simulink model "lab07"  (Simulink 10.3)
settings: Solver=FixedStepAuto  StartTime=0.0  StopTime=2.5  FixedStep=0.001768  RelTol=1e-3
values from neighbouring files (symbols this model uses):
  D = 0    [lab03.mat]    (also in lab04.mat; lab05.mat; lab07.mat; matlab.mat)
  k_d = 0.00416035381008    [lab03.mat]    (also in lab04.mat = 0.00114359359927; lab05.mat = 0.00883154670201; lab06.mat = 0.05; lab07.mat = 0.00883154670201)
  k_p = 2    [lab02.mat]    (also in lab03.mat = 0.256097247605; lab04.mat = 0.137612608424; lab05.mat = 0.280842058008; lab06.mat = 0.012)
undefined symbols (not defined in the file or in its folder): D_n, N_1, N_2, N_n
settings Model: Creator=kisdev  LastModifiedBy=kisdev
settings SolverCC: AlgebraicLoopSolver=Auto
settings DataIOCC: SaveFormat=Dataset  SignalLoggingSaveFormat=Dataset  ReturnWorkspaceOutputs=on
settings OptimizationCC: ExpressionDepthLimit=128  LifeSpan=auto
settings DebuggingCC: UnderspecifiedInitializationDetection=Simplified  MergeDetectMultiDrivingBlocksExec=error  FcnCallInpInsideContextMsg=error  StateNameClashWarn=none  SFUnexpectedBacktrackingDiag=error  SFNoUnconditionalDefaultTransitionDiag=error  SFExecutionAtInitializationDiag=warning  SFMachineParentedDataDiag=error  ArithmeticOperatorsInVariantConditions=error
settings HardwareCC: ProdBitPerPointer=64  ProdBitPerSizeT=64  ProdBitPerPtrDiffT=64  ProdLargestAtomicFloat=Float  ProdIntDivRoundTo=Zero  ProdEndianess=LittleEndian  ProdWordSize=64  ProdHWDeviceType=Intel->x86-64 (Windows64)
settings ModelReferenceCC: PropagateSignalLabelsOutOfModel=on
settings SFSimCC: SimUseLocalCustomCode=on  CustomCodeUndefinedFunction=FilterOut
settings RTWCC: RTWUseLocalCustomCode=on
settings CodeAppCC: StateflowObjectComments=off
settings GRTTargetCC: TargetLangStandard=C99 (ISO)  CombineOutputUpdateFcns=on  GRTInterface=off
settings ConfigComp: CovMetricSettings=dwe  CovSaveCumulativeToWorkspaceVar=off  CovSaveSingleToWorkspaceVar=off  CovExternalEMLEnable=on

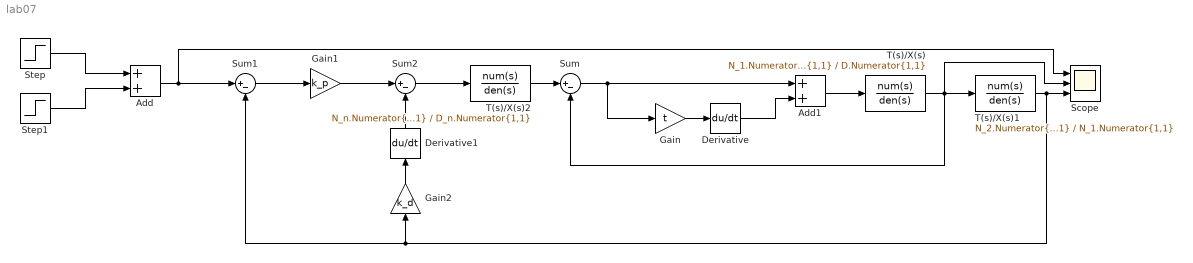
== system lab07 ==
  Add : Sum
  Add1 : Sum
  Derivative : Derivative
  Derivative1 : Derivative
  Gain : Gain  Gain=t
  Gain1 : Gain  Gain=k_p
  Gain2 : Gain  Gain=k_d
  Scope : Scope  NumInputPorts=3
  Step : Step  Time=0  After=500  SampleTime=0
  Step1 : Step  Time=10  After=-500  SampleTime=0
  Sum : Sum  Inputs=|+-
  Sum1 : Sum  Inputs=|+-
  Sum2 : Sum  Inputs=|+-
  T(s)/X(s) : TransferFcn  Numerator=N_1.Numerator{1,1}  Denominator=D.Numerator{1,1}
  T(s)/X(s)1 : TransferFcn  Numerator=N_2.Numerator{1,1}  Denominator=N_1.Numerator{1,1}
  T(s)/X(s)2 : TransferFcn  Numerator=N_n.Numerator{1,1}  Denominator=D_n.Numerator{1,1}
  wires:
  Step/1 -> Add/1
  Step1/1 -> Add/2
  T(s)/X(s)/1 -> Scope/2, T(s)/X(s)1/1, Sum/2
  Gain/1 -> Derivative/1
  Add1/1 -> T(s)/X(s)/1
  Derivative/1 -> Add1/2
  Sum/1 -> Gain/1, Add1/1
  Add/1 -> Sum1/1, Scope/1
  T(s)/X(s)1/1 -> Gain2/1, Sum1/2, Scope/3
  T(s)/X(s)2/1 -> Sum/1
  Gain1/1 -> Sum2/1
  Sum1/1 -> Gain1/1
  Sum2/1 -> T(s)/X(s)2/1
  Gain2/1 -> Derivative1/1
  Derivative1/1 -> Sum2/2
